simulink model "controllab5"  (R2015b)
settings: Solver=VariableStepAuto  StartTime=0.0  StopTime=1000  RelTol=1e-3
settings Model: Creator=BLUE COM  LastModifiedBy=BLUE COM

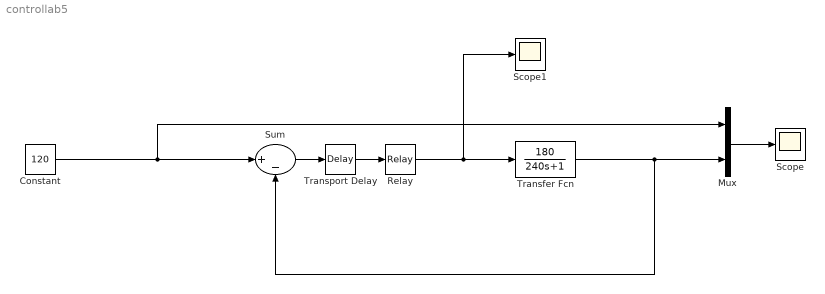
== system controllab5 ==
  Constant : Constant  Value=120
  Mux : Mux  Inputs=2
  Relay : Relay  OnSwitchValue=10  OffSwitchValue=-10
  Scope : Scope
  Scope1 : Scope
  Sum : Sum  Inputs=|+-
  Transfer Fcn : TransferFcn  Numerator=[180]  Denominator=[240 1]
  Transport Delay : TransportDelay  DelayTime=30
  wires:
  Mux/1 -> Scope/1
  Relay/1 -> Scope1/1, Transfer Fcn/1
  Sum/1 -> Transport Delay/1
  Transport Delay/1 -> Relay/1
  Transfer Fcn/1 -> Sum/2, Mux/2
  Constant/1 -> Mux/1, Sum/1
